simulink library "peripheral_utilities"  (R2022b)
settings: Solver=VariableStepAuto  StartTime=0.0  StopTime=10.0  RelTol=1e-3
libraries: simulink x3, spsCurrentMeasurementLib x1, spsVoltageMeasurementLib x1
settings Model: Creator=Javnson  LastModifiedBy=Javnson

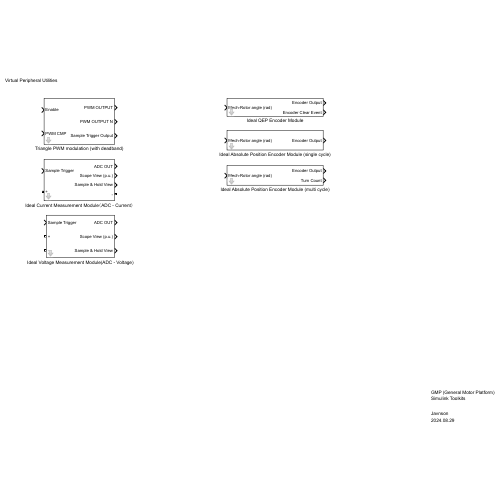
[thumbnail: Simulink's stored preview of the top-level diagram]
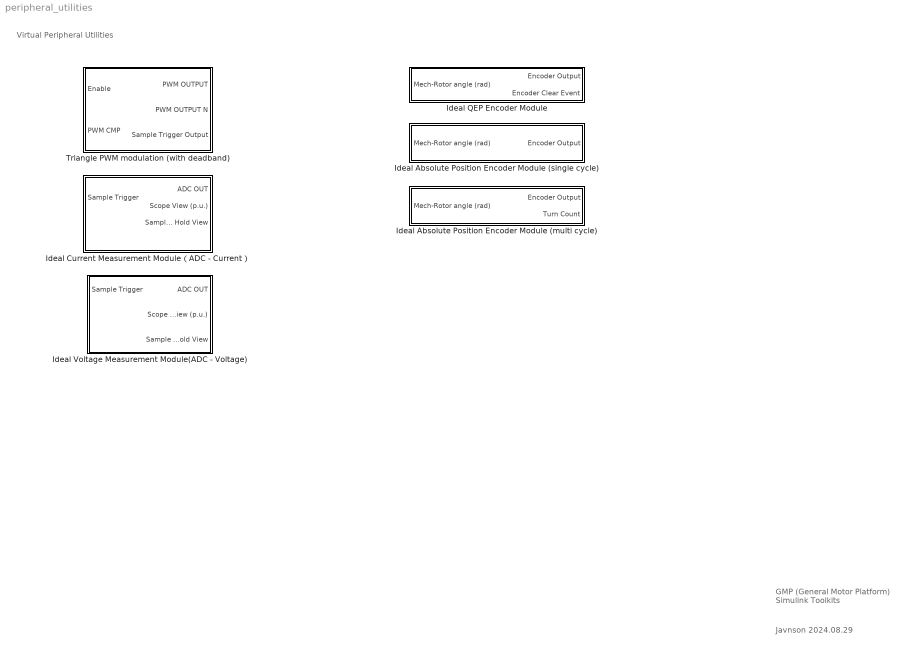
== system peripheral_utilities ==
  note: Virtual Peripheral Utilities
  note: GMP (General Motor Platform)
      | Simulink Toolkits
  note: Javnson
      | 2024.08.29
  Ideal Absolute Position Encoder Module (multi cycle) : Subsystem  mask{ENCODER_BIT=17}
      mask DialogControl DescGroupVar Prompt: Ideal Absolute Position Encoder Module (multi cycle)
      mask DialogControl DescTextVar Prompt: Avsolute Encoder transfer a motor mechanical angle (thetam, rad) to Absolute Encoder result. Generally, an absolute encoder has 17-bits or 23-bits resolution results.
      mask DialogControl ParameterGroupVar Prompt: 参数
      mask DialogControl Control2 Prompt: Absolute Encoder Resolution (bits):
  Ideal Absolute Position Encoder Module (single cycle) : Subsystem  mask{ENCODER_BIT=17}
      mask DialogControl DescGroupVar Prompt: Ideal Absolute Position Encoder Module (single cycle)
      mask DialogControl DescTextVar Prompt: Avsolute Encoder transfer a motor angle (thetam, rad) to Absolute Encoder result. Generally, an absolute encoder has 17-bits or 23-bits resolution results.
      mask DialogControl ParameterGroupVar Prompt: 参数
      mask DialogControl Control2 Prompt: Absolute Encoder Resolution (bits):
  Ideal Current Measurement Module（ADC - Current） : Subsystem  mask{ADC_GAIN=0.5, ADC_BIT=16, ADC_REFERENCE=20.0, ADC_BIAS=5, ADC_INIT=0}
      mask DialogControl DescGroupVar Prompt: Current Sample ADC Model 1
      mask DialogControl DescTextVar Prompt: This is a ideal Current Measurement Module. This module enable a bias and a gain, and finally output a ADC result.
      mask DialogControl Control8 Prompt: ADC(p.u.) = (real_current * ADC_GAIN + ADC_BIAS)/ADC_REFERENCE
      mask DialogControl ParameterGroupVar Prompt: 参数
      mask DialogControl Control7 Prompt: ADC Current Gain (Scale Factor):
      mask DialogControl Control2 Prompt: ADC resolution:
      mask DialogControl Control4 Prompt: ADC reference Current(A)
      mask DialogControl Control5 Prompt: ADC Bias Current(A)
      mask DialogControl Control6 Prompt: ADC initial Current Output(A)
  Ideal QEP Encoder Module : Subsystem  mask{QEP_LINE=2000}
      mask DialogControl DescGroupVar Prompt: Ideal QEP Encoder Module
      mask DialogControl DescTextVar Prompt: QEP encoder transfer a motor mechanical angle (thetam, rad) to QEP encoder results. The maximum output is 4 * QEP_LINE and generate a reseet event each round.
      mask DialogControl ParameterGroupVar Prompt: 参数
      mask DialogControl Control3 Prompt: QEP encoder lines count:
  Ideal Voltage Measurement Module(ADC - Voltage) : Subsystem  mask{ADC_BIAS=0, ADC_GAIN=1/10, ADC_BIT=16, ADC_REFERENCE=3, ADC_INIT=0}
      mask DialogControl DescGroupVar Prompt: Voltage Sample ADC Model
      mask DialogControl DescTextVar Prompt: This is a ideal Voltage Measurement Module.
      mask DialogControl Control2 Prompt: ADC(p.u.) = (real_voltage * ADC_GAIN + ADC_BIAS)/ADC_REFERENCE
      mask DialogControl ParameterGroupVar Prompt: Parameters:
      mask DialogControl Control4 Prompt: ADC Voltage Gain (Scale Factor):
      mask DialogControl Control5 Prompt: ADC resolution:
      mask DialogControl Control6 Prompt: ADC reference Voltage(V)
      mask DialogControl Control8 Prompt: ADC Bias Voltage(V)
      mask DialogControl Control7 Prompt: ADC Initial Voltage Output (V):
  Triangle PWM modulation (with deadband) : Subsystem  mask{fswitch=10e3, CMP_MAX=2000, Deadband_Upper=200, Deadband_upper_us=0, Deadband_Lower=100}
      mask prompts: Deadband_upper_us "Deadband Time: (μs)"
      mask init:
      | %dead_cmp_upper_param = get_pram(gcb, 'Deadband_Upper');
      mask Callback Deadband_Upper: %dead_cmp_param = get_param('DEADBAND_CMP','Value');
      mask DialogControl DescGroupVar Prompt: PWM Modulator
      mask DialogControl DescTextVar Prompt: PWM Modulator. Input PWM compare register value, output ADC trigger signal, PWM output and negtive PWM output.
      mask DialogControl ParameterGroupVar Prompt: 参数
      mask DialogControl Control2 Prompt: PWM Frequency (Hz) :
      mask DialogControl Control4 Prompt: Full Scale PWM Compare value:
      mask DialogControl Control5 Prompt: (whole period is 2 * CMP_MAX ticks)
      mask DialogControl Control3 Prompt: Deadband Range Set (CMP Value):
      mask DialogControl Control6 Prompt: Single side deadband time: DEADBAND_CMP/2/CMP_MAX/fswitch

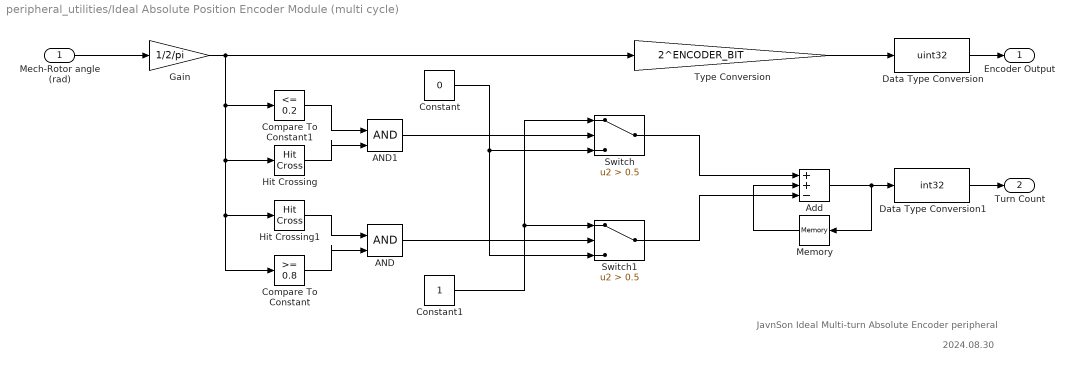
== system peripheral_utilities/Ideal Absolute Position Encoder Module (multi cycle) ==
  note: JavnSon Ideal Multi-turn Absolute Encoder peripheral
  note: 2024.08.30
  Mech-Rotor angle (rad) : Inport
  AND : Logic  IconShape=distinctive  AllPortsSameDT=off  OutDataTypeStr=boolean
  AND1 : Logic  IconShape=distinctive  AllPortsSameDT=off  OutDataTypeStr=boolean
  Add : Sum  Inputs=++-
  Compare To Constant : simulink/Logic and Bit Operations/Compare To Constant  relop=>=  const=0.8  OutDataTypeStr=boolean
  Compare To Constant1 : simulink/Logic and Bit Operations/Compare To Constant  relop=<=  const=0.2  OutDataTypeStr=boolean
  Constant : Constant  Value=0
  Constant1 : Constant
  Data Type Conversion : DataTypeConversion  OutDataTypeStr=uint32  SaturateOnIntegerOverflow=off  RndMeth=Floor
  Data Type Conversion1 : DataTypeConversion  OutDataTypeStr=int32  SaturateOnIntegerOverflow=off  RndMeth=Floor
  Gain : Gain  Gain=1/2/pi
  Hit Crossing : HitCross  HitCrossingOffset=0.5  HitCrossingDirection=falling
  Hit Crossing1 : HitCross  HitCrossingOffset=0.5  HitCrossingDirection=rising
  Memory : Memory
  Switch : Switch  Criteria=u2 > Threshold  Threshold=0.5  SaturateOnIntegerOverflow=off  InputSameDT=off
  Switch1 : Switch  Criteria=u2 > Threshold  Threshold=0.5  SaturateOnIntegerOverflow=off  InputSameDT=off
  Type Conversion : Gain  Gain=2^ENCODER_BIT
  Encoder Output : Outport
  Turn Count : Outport  Port=2
  wires:
  Gain/1 -> Compare To Constant1/1, Hit Crossing/1, Compare To Constant/1, Hit Crossing1/1, Type Conversion/1
  Type Conversion/1 -> Data Type Conversion/1
  Data Type Conversion/1 -> Encoder Output/1
  Mech-Rotor angle (rad)/1 -> Gain/1
  Memory/1 -> Add/2
  Add/1 -> Data Type Conversion1/1, Memory/1
  Switch/1 -> Add/1
  Hit Crossing1/1 -> AND/1
  Data Type Conversion1/1 -> Turn Count/1
  Switch1/1 -> Add/3
  Compare To Constant/1 -> AND/2
  AND/1 -> Switch1/2
  Hit Crossing/1 -> AND1/2
  Compare To Constant1/1 -> AND1/1
  AND1/1 -> Switch/2
  Constant1/1 -> Switch1/1, Switch/1
  Constant/1 -> Switch1/3, Switch/3

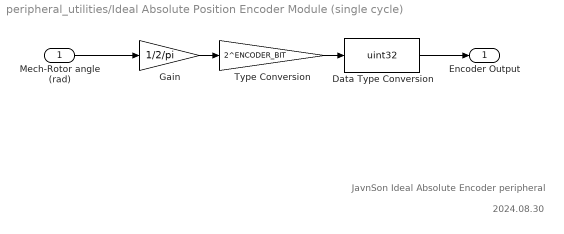
== system peripheral_utilities/Ideal Absolute Position Encoder Module (single cycle) ==
  note: 2024.08.30
  note: JavnSon Ideal Absolute Encoder peripheral
  Mech-Rotor angle (rad) : Inport
  Data Type Conversion : DataTypeConversion  OutDataTypeStr=uint32  SaturateOnIntegerOverflow=off  RndMeth=Floor
  Gain : Gain  Gain=1/2/pi
  Type Conversion : Gain  Gain=2^ENCODER_BIT
  Encoder Output : Outport
  wires:
  Gain/1 -> Type Conversion/1
  Type Conversion/1 -> Data Type Conversion/1
  Data Type Conversion/1 -> Encoder Output/1
  Mech-Rotor angle (rad)/1 -> Gain/1

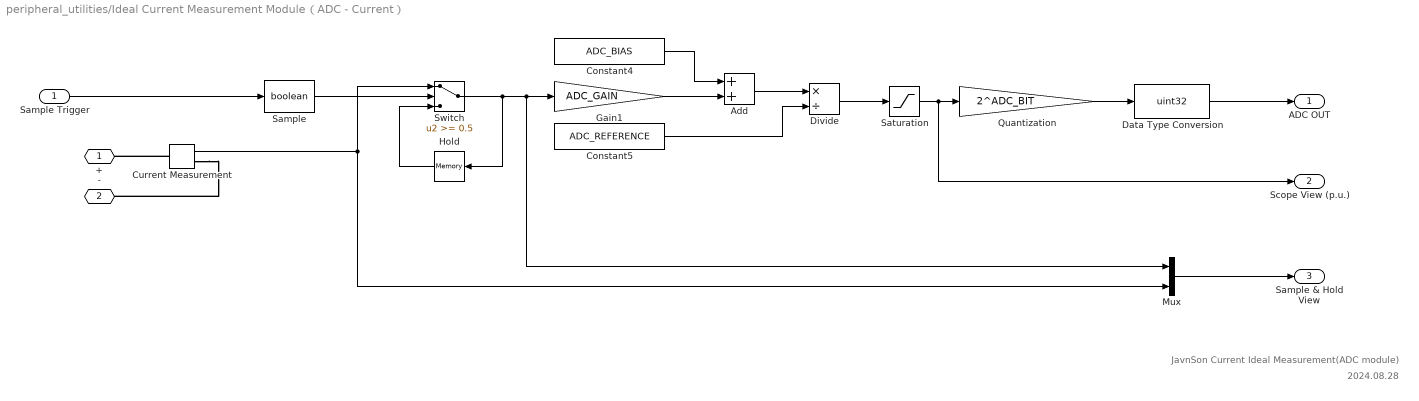
== system peripheral_utilities/Ideal Current Measurement Module（ADC - Current） ==
  note: JavnSon Current Ideal Measurement(ADC module)
  note: 2024.08.28
  Sample Trigger : Inport
  Add : Sum
  Constant4 : Constant  Value=ADC_BIAS
  Constant5 : Constant  Value=ADC_REFERENCE
  Current Measurement : spsCurrentMeasurementLib/Current Measurement  PhasorSimulation=off  OutputType=Complex  PSBequivalent=0
  Data Type Conversion : DataTypeConversion  OutDataTypeStr=uint32  ConvertRealWorld=Stored Integer (SI)  SaturateOnIntegerOverflow=off  RndMeth=Floor
  Divide : Product  Inputs=*/
  Gain1 : Gain  Gain=ADC_GAIN
  Hold : Memory  InitialCondition=ADC_INIT  LinearizeAsDelay=on
  Mux : Mux  Inputs=2
  Quantization : Gain  Gain=2^ADC_BIT
  Sample : DataTypeConversion  OutDataTypeStr=boolean  SaturateOnIntegerOverflow=off  RndMeth=Floor
  Saturation : Saturate  UpperLimit=1  LowerLimit=0
  Switch : Switch  Threshold=0.5
  + : PMIOPort  Side=Left
  - : PMIOPort  Port=2  Side=Right
  ADC OUT : Outport
  Scope View (p.u.) : Outport  Port=2
  Sample & Hold View : Outport  Port=3
  wires:
  Constant5/1 -> Divide/2
  Quantization/1 -> Data Type Conversion/1
  Sample/1 -> Switch/2
  Add/1 -> Divide/1
  Sample Trigger/1 -> Sample/1
  Data Type Conversion/1 -> ADC OUT/1
  Hold/1 -> Switch/3
  Current Measurement/1 -> Mux/2, Switch/1
  Constant4/1 -> Add/1
  Switch/1 -> Hold/1, Mux/1, Gain1/1
  Gain1/1 -> Add/2
  Saturation/1 -> Scope View (p.u.)/1, Quantization/1
  Divide/1 -> Saturation/1
  Mux/1 -> Sample & Hold View/1
  connections:
  Current Measurement/LConn1 -- +/RConn1
  Current Measurement/RConn1 -- -/RConn1

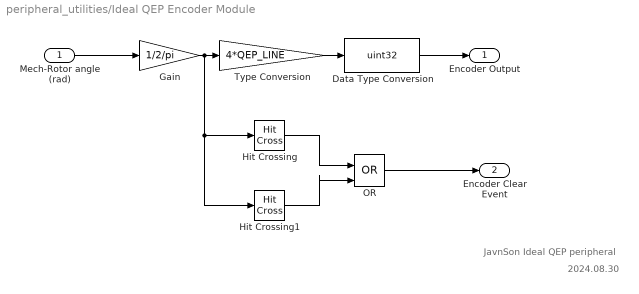
== system peripheral_utilities/Ideal QEP Encoder Module ==
  note: JavnSon Ideal QEP peripheral
  note: 2024.08.30
  Mech-Rotor angle (rad) : Inport
  Data Type Conversion : DataTypeConversion  OutDataTypeStr=uint32  SaturateOnIntegerOverflow=off  RndMeth=Floor
  Gain : Gain  Gain=1/2/pi
  Hit Crossing : HitCross  HitCrossingDirection=rising
  Hit Crossing1 : HitCross  HitCrossingOffset=1  HitCrossingDirection=falling
  OR : Logic  Operator=OR  IconShape=distinctive  AllPortsSameDT=off  OutDataTypeStr=boolean
  Type Conversion : Gain  Gain=4*QEP_LINE
  Encoder Output : Outport
  Encoder Clear Event : Outport  Port=2
  wires:
  Mech-Rotor angle (rad)/1 -> Gain/1
  Data Type Conversion/1 -> Encoder Output/1
  Type Conversion/1 -> Data Type Conversion/1
  Gain/1 -> Hit Crossing1/1, Hit Crossing/1, Type Conversion/1
  OR/1 -> Encoder Clear Event/1
  Hit Crossing/1 -> OR/1
  Hit Crossing1/1 -> OR/2

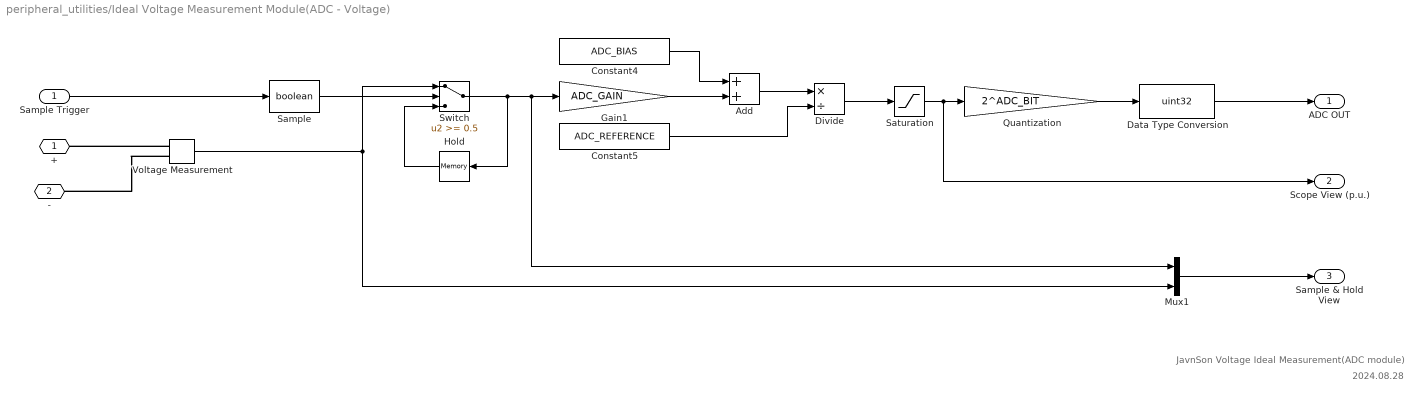
== system peripheral_utilities/Ideal Voltage Measurement Module(ADC - Voltage) ==
  note: JavnSon Voltage Ideal Measurement(ADC module)
  note: 2024.08.28
  Sample Trigger : Inport
  Add : Sum
  Constant4 : Constant  Value=ADC_BIAS
  Constant5 : Constant  Value=ADC_REFERENCE
  Data Type Conversion : DataTypeConversion  OutDataTypeStr=uint32  ConvertRealWorld=Stored Integer (SI)  SaturateOnIntegerOverflow=off  RndMeth=Floor
  Divide : Product  Inputs=*/
  Gain1 : Gain  Gain=ADC_GAIN
  Hold : Memory  InitialCondition=ADC_INIT  LinearizeAsDelay=on
  Mux1 : Mux  Inputs=2
  Quantization : Gain  Gain=2^ADC_BIT
  Sample : DataTypeConversion  OutDataTypeStr=boolean  SaturateOnIntegerOverflow=off  RndMeth=Floor
  Saturation : Saturate  UpperLimit=1  LowerLimit=0
  Switch : Switch  Threshold=0.5
  Voltage Measurement : spsVoltageMeasurementLib/Voltage Measurement  PhasorSimulation=off  OutputType=Complex  PSBequivalent=0
  + : PMIOPort  Side=Left
  - : PMIOPort  Port=2  Side=Left
  ADC OUT : Outport
  Scope View (p.u.) : Outport  Port=2
  Sample & Hold View : Outport  Port=3
  wires:
  Hold/1 -> Switch/3
  Switch/1 -> Hold/1, Mux1/1, Gain1/1
  Divide/1 -> Saturation/1
  Voltage Measurement/1 -> Mux1/2, Switch/1
  Saturation/1 -> Scope View (p.u.)/1, Quantization/1
  Constant4/1 -> Add/1
  Gain1/1 -> Add/2
  Sample Trigger/1 -> Sample/1
  Data Type Conversion/1 -> ADC OUT/1
  Mux1/1 -> Sample & Hold View/1
  Quantization/1 -> Data Type Conversion/1
  Constant5/1 -> Divide/2
  Add/1 -> Divide/1
  Sample/1 -> Switch/2
  connections:
  Voltage Measurement/LConn1 -- +/RConn1
  Voltage Measurement/LConn2 -- -/RConn1

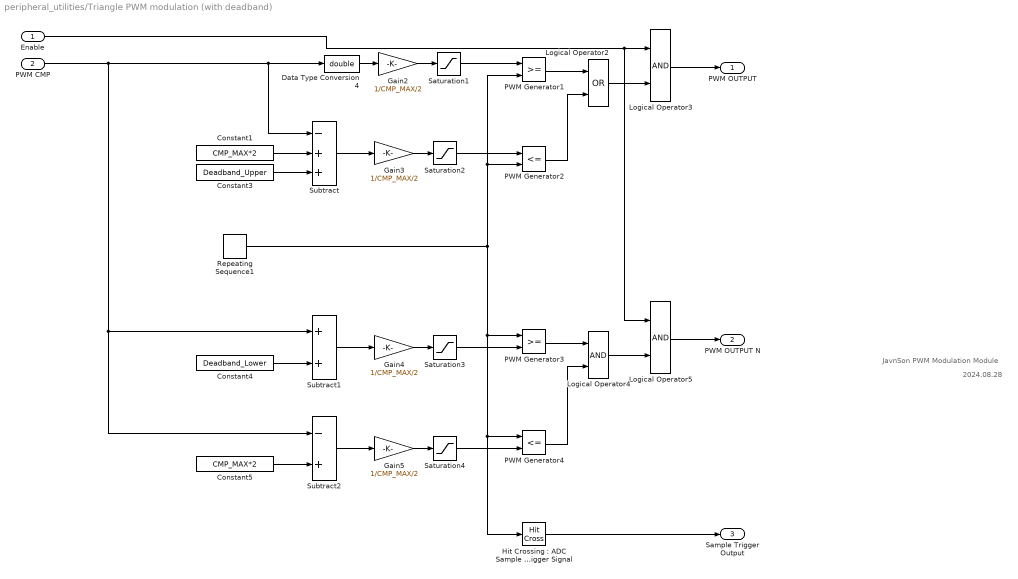
== system peripheral_utilities/Triangle PWM modulation (with deadband) ==
  note: 2024.08.28
  note: JavnSon PWM Modulation Module
  Enable : Inport
  PWM CMP : Inport  Port=2
  Constant1 : Constant  Value=CMP_MAX*2
  Constant3 : Constant  Value=Deadband_Upper
  Constant4 : Constant  Value=Deadband_Lower
  Constant5 : Constant  Value=CMP_MAX*2
  Data Type Conversion4 : DataTypeConversion  OutDataTypeStr=double  SaturateOnIntegerOverflow=off  RndMeth=Floor
  Gain{2..5} (4 alike) : Gain  Gain=1/CMP_MAX/2
  Hit Crossing：ADC Sample Trigger Signal : HitCross  HitCrossingOffset=0.5  HitCrossingDirection=rising
  Logical Operator2 : Logic  Operator=OR  AllPortsSameDT=off  OutDataTypeStr=boolean
  Logical Operator3 : Logic  AllPortsSameDT=off  OutDataTypeStr=boolean
  Logical Operator4 : Logic  AllPortsSameDT=off  OutDataTypeStr=boolean
  Logical Operator5 : Logic  AllPortsSameDT=off  OutDataTypeStr=boolean
  PWM Generator1 : RelationalOperator  OutDataTypeStr=boolean  InputSameDT=off
  PWM Generator2 : RelationalOperator  Operator=<=  OutDataTypeStr=boolean  InputSameDT=off
  PWM Generator3 : RelationalOperator  OutDataTypeStr=boolean  InputSameDT=off
  PWM Generator4 : RelationalOperator  Operator=<=  OutDataTypeStr=boolean  InputSameDT=off
  Repeating Sequence1 : simulink/Sources/Repeating Sequence  rep_seq_t=[0, 1/2/fswitch, 1/fswitch ]  rep_seq_y=[0, 0.5, 1]
  Saturation{1..4} (4 alike) : Saturate  UpperLimit=1  LowerLimit=0
  Subtract : Sum  Inputs=-++
  Subtract1 : Sum
  Subtract2 : Sum  Inputs=-+
  PWM OUTPUT : Outport
  PWM OUTPUT N : Outport  Port=2
  Sample Trigger Output : Outport  Port=3
  wires:
  PWM CMP/1 -> Subtract2/1, Subtract1/1, Subtract/1, Data Type Conversion4/1
  Data Type Conversion4/1 -> Gain2/1
  Gain2/1 -> Saturation1/1
  Saturation1/1 -> PWM Generator1/1
  PWM Generator1/1 -> Logical Operator2/1
  Logical Operator2/1 -> Logical Operator3/2
  Constant1/1 -> Subtract/2
  Constant3/1 -> Subtract/3
  PWM Generator2/1 -> Logical Operator2/2
  Gain3/1 -> Saturation2/1
  Subtract/1 -> Gain3/1
  Saturation2/1 -> PWM Generator2/1
  Constant4/1 -> Subtract1/2
  Gain4/1 -> Saturation3/1
  Subtract1/1 -> Gain4/1
  Saturation3/1 -> PWM Generator3/2
  PWM Generator3/1 -> Logical Operator4/1
  Constant5/1 -> Subtract2/2
  Saturation4/1 -> PWM Generator4/2
  Gain5/1 -> Saturation4/1
  Subtract2/1 -> Gain5/1
  PWM Generator4/1 -> Logical Operator4/2
  Logical Operator4/1 -> Logical Operator5/2
  Repeating Sequence1/1 -> PWM Generator2/2, PWM Generator1/2, PWM Generator3/1, Hit Crossing：ADC Sample Trigger Signal/1, PWM Generator4/1
  Enable/1 -> Logical Operator5/1, Logical Operator3/1
  Logical Operator5/1 -> PWM OUTPUT N/1
  Logical Operator3/1 -> PWM OUTPUT/1
  Hit Crossing：ADC Sample Trigger Signal/1 -> Sample Trigger Output/1
